simulink model "X_k"  (R2024b)
settings: Solver=FixedStepAuto  StartTime=0.0  StopTime=10.0  FixedStep=1  RelTol=1e-3
undefined symbols (not defined in the file): D
settings Model: Creator=54238  LastModifiedBy=54238

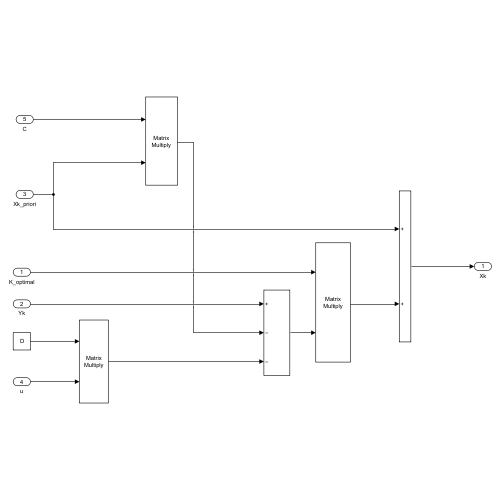
[thumbnail: Simulink's stored preview of the top-level diagram]
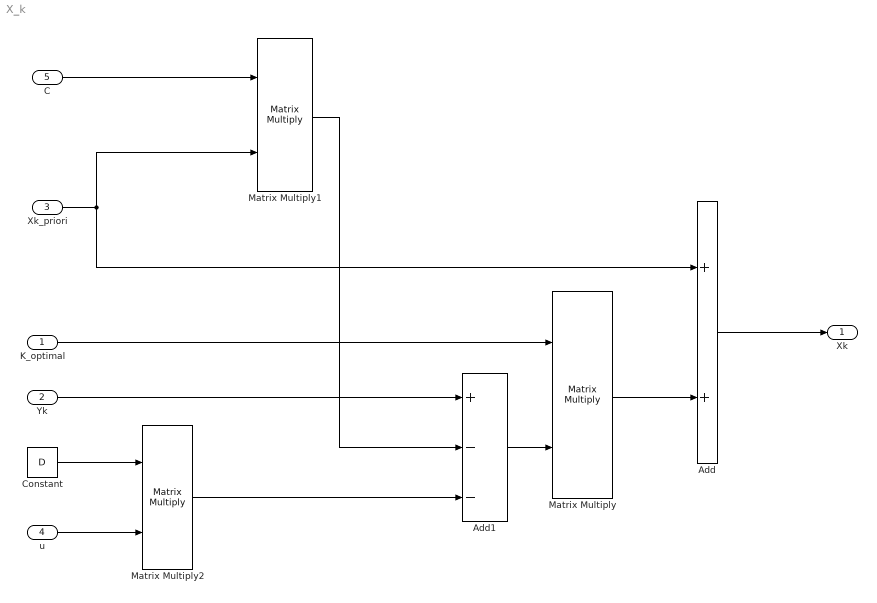
== system X_k ==
  K_optimal : Inport  PortDimensions=[4,2]
  Yk : Inport  Port=2  PortDimensions=[2,1]
  Xk_priori : Inport  Port=3  PortDimensions=[4,1]
  u : Inport  Port=4  PortDimensions=[2,1]
  C : Inport  Port=5  PortDimensions=[2,4]
  Add : Sum
  Add1 : Sum  Inputs=+--
  Constant : Constant  Value=D
  Matrix Multiply : Product  Multiplication=Matrix(*)
  Matrix Multiply1 : Product  Multiplication=Matrix(*)
  Matrix Multiply2 : Product  Multiplication=Matrix(*)
  Xk : Outport  PortDimensions=[4,1]
  wires:
  Xk_priori/1 -> Matrix Multiply1/2, Add/1
  K_optimal/1 -> Matrix Multiply/1
  C/1 -> Matrix Multiply1/1
  Yk/1 -> Add1/1
  Matrix Multiply2/1 -> Add1/3
  Matrix Multiply1/1 -> Add1/2
  Constant/1 -> Matrix Multiply2/1
  u/1 -> Matrix Multiply2/2
  Add1/1 -> Matrix Multiply/2
  Matrix Multiply/1 -> Add/2
  Add/1 -> Xk/1
